simulink model "WindPrototipeN"  (R2019b)
settings: Solver=ode23s  StartTime=0.0  StopTime=Ts  FixedStep=2  RelTol=5
values from neighbouring files (symbols this model uses):
  c1 = 0.51763    [matlab.mat]
  c2 = 116    [matlab.mat]
  c3 = 0.4    [matlab.mat]
  c4 = 5    [matlab.mat]
  c5 = 21    [matlab.mat]
  c6 = 0.006795    [matlab.mat]
  Tp = 2e-05    [matlab.mat]
undefined symbols (not defined in the file or in its folder): Cogent, DiscIntNeverNeededParam, Ion, Kepware, Lithium, localhost, sigbuilder_block
libraries: powerlib x266, powerlib_extras x83, simulink x30, powerlib_meascontrol x13, opclib x11, sldrtlib x8, electricdrivelib x3
(part 7 of 9)

== system WindPrototipeN/Дом 2/ВЕТРОТУРБИНА И ГЕНЕРАТОР1/Модель турбины ==
  Generator speed (pu) : Inport
  Pitch angle (deg) : Inport  Port=2
  Wind speed (m/s) : Inport  Port=3
  Air density : Inport  Port=4
  1/cp_nom : Gain  Gain=1/cp_nom  SaturateOnIntegerOverflow=on  OutDataTypeStr=Inherit: Same as input  ParamDataTypeStr=Inherit: Same as input
  1/wind_base : Gain  Gain=1/wind_base  SaturateOnIntegerOverflow=on  OutDataTypeStr=Inherit: Same as input  ParamDataTypeStr=Inherit: Same as input
  Avoid division by zero : Saturate  UpperLimit=1e6  LowerLimit=1e-6
  "Avoid division by zero " : Saturate  UpperLimit=1e6  LowerLimit=1e-6
  Gain : Gain  Gain=-1  SaturateOnIntegerOverflow=on  OutDataTypeStr=Inherit: Same as input  ParamDataTypeStr=Inherit: Same as input
  Product : Product  Inputs=/*  SaturateOnIntegerOverflow=on  OutDataTypeStr=Inherit: Same as first input
  "Product " : Product  Inputs=3  SaturateOnIntegerOverflow=on  OutDataTypeStr=Inherit: Same as first input
  Product2 : Product  Inputs=*/  SaturateOnIntegerOverflow=on  InputSameDT=on  OutDataTypeStr=Inherit: Same as first input
  Saturation1 : Saturate  UpperLimit=inf  LowerLimit=1e-6
  Scope : Scope
  cp(lambda,beta) : Subsystem
  lambda_nom : Gain  Gain=lambda_nom  SaturateOnIntegerOverflow=on  OutDataTypeStr=Inherit: Same as input  ParamDataTypeStr=Inherit: Same as input
  pu->pu : Gain  Gain=P_wind_base*Pnom/Pelec_base  SaturateOnIntegerOverflow=on  OutDataTypeStr=Inherit: Same as input  ParamDataTypeStr=Inherit: Same as input
  "pu->pu " : Gain  Gain=1/speed_nom  SaturateOnIntegerOverflow=on  OutDataTypeStr=Inherit: Same as input  ParamDataTypeStr=Inherit: Same as input
  wind_speed^3 : Fcn  Expr=u(1)^3
  Tm (pu) : Outport  VectorParamsAs1DForOutWhenUnconnected=off
  wires:
  Pitch angle (deg)/1 -> cp(lambda,beta)/2(beta)
  pu->pu/1 -> Product2/1
  cp(lambda,beta)/1(cp) -> 1/cp_nom/1
  wind_speed^3/1 -> "Product "/1  "Pwind_pu"
  Product2/1 -> Gain/1
  Avoid division by zero/1 -> Product2/2
  Wind speed (m/s)/1 -> 1/wind_base/1
  Gain/1 -> Tm (pu)/1
  Generator speed (pu)/1 -> Avoid division by zero/1, "pu->pu "/1
  "Product "/1 -> pu->pu/1  "Pm_pu"
  lambda_nom/1 -> Saturation1/1  "lambda"
  1/cp_nom/1 -> "Product "/2  "cp_pu"
  Saturation1/1 -> cp(lambda,beta)/1(lambda), Scope/1
  Product/1 -> lambda_nom/1  "lambda_pu"
  1/wind_base/1 -> wind_speed^3/1, "Avoid division by zero "/1  "wind_speed_pu"
  "Avoid division by zero "/1 -> Product/1
  "pu->pu "/1 -> Product/2
  Air density/1 -> "Product "/3

== system WindPrototipeN/Дом 2/ВЕТРОТУРБИНА И ГЕНЕРАТОР1/Расчет номинального момента ==
  ПВ : Inport
  ОП : Inport  Port=2
  Base Torque : Product  Inputs=*/  RndMeth=Zero
  Base_torque_ : Display
  Constant1 : Constant  Value=8500
  Constant2 : Constant  Value=152.89
  Manual Switch1 : ManualSwitch  CurrentSetting=0
  Mux : Mux  Inputs=6
  Корректирующий коэффициент1 : Constant  Value=.0000133
  Коэффициент эффективности : Constant  Value=.43
  Номинальная мощность Вт : Constant  Value=2200
  Номинальная скорость ветра : Constant  Value=10
  Расчет номинального момента : Fcn  Expr=1/2*u(1)*u(2)*u(3)*u(4)^3*u(5)*u(6)
  Номинальный момент : Outport  VectorParamsAs1DForOutWhenUnconnected=off
  r : Outport  Port=2  VectorParamsAs1DForOutWhenUnconnected=off
  wires:
  Constant1/1 -> Base Torque/1
  ОП/1 -> Mux/2
  Расчет номинального момента/1 -> Manual Switch1/2, Base_torque_/1
  Коэффициент эффективности/1 -> Mux/3
  Номинальная скорость ветра/1 -> Mux/4
  Корректирующий коэффициент1/1 -> Mux/5
  Mux/1 -> Расчет номинального момента/1
  Номинальная мощность Вт/1 -> Mux/6
  Constant2/1 -> Manual Switch1/1
  Manual Switch1/1 -> r/1, Base Torque/2
  ПВ/1 -> Mux/1
  Base Torque/1 -> Номинальный момент/1

== system WindPrototipeN/Дом 2/ВХОДНЫЕ ЗНАЧЕНИЯ ДЛЯ ВЭУ1/Задание кривой скорости ==
  Demux : Demux  Tag=STV Demux  Outputs=1
  FromWs : FromWorkspace  Tag=STV FromWs  VariableName=tuvar  SampleTime=0
      SigBuilderData=|
      | common.afterFinalStr = 'Extrapolate'
      | common.sampleTime = 0
      | dataSet.timeRange = [0 15]
      | dataSet.name = 'Group 1'
      | sbobj.Groups.Name = 'Group 1'
      | sbobj.Groups.Signals.Name = 'Signal 1'
      | sbobj.Groups.Signals.XData = [0 1.5 2 2.5 3 4 4 5 5 7 8 9 11 15]
      | sbobj.Groups.Signals.YData = [8.31 8.86 8.78 8.7 7.74 8.06 8.12 7.62 7.9 7.5 7.18 7.84 7.32 6.54]
      | sbobj.Groups.TimeRange = [0 15]
  Signal 1 : Outport  Tag=STV Outport  VectorParamsAs1DForOutWhenUnconnected=off
  wires:
  Demux/1 -> Signal 1/1
  FromWs/1 -> Demux/1

== system WindPrototipeN/Дом 2/ВХОДНЫЕ ЗНАЧЕНИЯ ДЛЯ ВЭУ1/Задание кривой скорости1 ==
  Demux : Demux  Tag=STV Demux  Outputs=1
  FromWs : FromWorkspace  Tag=STV FromWs  VariableName=tuvar  SampleTime=0
      SigBuilderData=|
      | common.afterFinalStr = 'Extrapolate'
      | common.sampleTime = 0
      | dataSet.timeRange = [0 15]
      | dataSet.name = 'Group 1'
      | sbobj.Groups.Name = 'Group 1'
      | sbobj.Groups.Signals.Name = 'Signal 1'
      | sbobj.Groups.Signals.XData = [0 1.5 2 2.5 3 4 5 7 8 9 11 15]
      | sbobj.Groups.Signals.YData = [11.1 11.6 11.9 12.12 11.88 11.32 11.98 11.6 12 11.56 11.26 12]
      | sbobj.Groups.TimeRange = [0 15]
  Signal 1 : Outport  Tag=STV Outport  VectorParamsAs1DForOutWhenUnconnected=off
  wires:
  Demux/1 -> Signal 1/1
  FromWs/1 -> Demux/1

== system WindPrototipeN/Дом 2/ВХОДНЫЕ ЗНАЧЕНИЯ ДЛЯ СЭС1/Задание кривой солнечной радиации ==
  Demux : Demux  Tag=STV Demux
  FromWs : FromWorkspace  Tag=STV FromWs  VariableName=tuvar  SampleTime=0
      SigBuilderData=|
      | common.afterFinalStr = 'Extrapolate'
      | common.sampleTime = 0
      | dataSet.timeRange = [0 15]
      | dataSet.name = 'Group 1'
      | sbobj.Groups.Name = 'Group 1'
      | sbobj.Groups.Signals(1).Name = 'Signal 1'
      | sbobj.Groups.Signals(1).XData = [0 1 5 8 9 15]
      | sbobj.Groups.Signals(1).YData = [0 115 210 528 230 0]
      | sbobj.Groups.Signals(2).Name = 'Signal 2'
      | sbobj.Groups.Signals(2).XData = [0 2 2 3 3 15]
      | sbobj.Groups.Signals(2).YData = [0 0 1 1 0 0]
      | sbobj.Groups.Signals(3).Name = 'Signal 3'
      | sbobj.Groups.Signals(3).XData = [0 2.5 2.5 15]
      | sbobj.Groups.Signals(3).YData = [0 0 1 1]
      | sbobj.Groups.Signals(4).Name = 'Signal 4'
      | sbobj.Groups.Signals(4).XData = [0 2.5 2.5 15]
      | sbobj.Groups.Signals(4).YData = [0 0 1 1]
      | sbobj.Groups.TimeRange = [0 15]
  Signal 1 : Outport  Tag=STV Outport  VectorParamsAs1DForOutWhenUnconnected=off
  Signal 2 : Outport  Tag=STV Outport  Port=2
  Signal 3 : Outport  Tag=STV Outport  Port=3
  Signal 4 : Outport  Tag=STV Outport  Port=4
  wires:
  Demux/1 -> Signal 1/1
  FromWs/1 -> Demux/1
  Demux/2 -> Signal 2/1
  Demux/3 -> Signal 3/1
  Demux/4 -> Signal 4/1

== system WindPrototipeN/Дом 2/КОНТРОЛЛЕР БАТАРЕИ/Discrete PI Controller ==
  Error : Inport
  Discrete-Time Integrator : DiscreteIntegrator  InitialCondition=Init  SampleTime=Ts  LimitOutput=on  UpperSaturationLimit=UpperLimit  LowerSaturationLimit=LowerLimit  ICPrevOutput=DiscIntNeverNeededParam  ICPrevScaledInput=DiscIntNeverNeededParam
  Kp4 : Gain  Gain=Kp  SaturateOnIntegerOverflow=on  OutDataTypeStr=Inherit: Same as input  ParamDataTypeStr=Inherit: Same as input
  Kp5 : Gain  Gain=Ki  SaturateOnIntegerOverflow=on  OutDataTypeStr=Inherit: Same as input  ParamDataTypeStr=Inherit: Same as input
  Saturation2 : Saturate  UpperLimit=UpperLimit  LowerLimit=LowerLimit
  Sum6 : Sum  SaturateOnIntegerOverflow=on  InputSameDT=on  OutDataTypeStr=Inherit: Same as first input
  Out : Outport  InitialOutput=0  VectorParamsAs1DForOutWhenUnconnected=off
  wires:
  Saturation2/1 -> Out/1
  Discrete-Time Integrator/1 -> Sum6/2
  Kp4/1 -> Sum6/1
  Kp5/1 -> Discrete-Time Integrator/1
  Sum6/1 -> Saturation2/1
  Error/1 -> Kp5/1, Kp4/1

== system WindPrototipeN/Дом 2/КОНТРОЛЛЕР БАТАРЕИ/Discrete PI Controller1 ==
  Error : Inport
  Discrete-Time Integrator : DiscreteIntegrator  InitialCondition=Init  SampleTime=Ts  LimitOutput=on  UpperSaturationLimit=UpperLimit  LowerSaturationLimit=LowerLimit  ICPrevOutput=DiscIntNeverNeededParam  ICPrevScaledInput=DiscIntNeverNeededParam
  Kp4 : Gain  Gain=Kp  SaturateOnIntegerOverflow=on  OutDataTypeStr=Inherit: Same as input  ParamDataTypeStr=Inherit: Same as input
  Kp5 : Gain  Gain=Ki  SaturateOnIntegerOverflow=on  OutDataTypeStr=Inherit: Same as input  ParamDataTypeStr=Inherit: Same as input
  Saturation2 : Saturate  UpperLimit=UpperLimit  LowerLimit=LowerLimit
  Sum6 : Sum  SaturateOnIntegerOverflow=on  InputSameDT=on  OutDataTypeStr=Inherit: Same as first input
  Out : Outport  InitialOutput=0  VectorParamsAs1DForOutWhenUnconnected=off
  wires:
  Saturation2/1 -> Out/1
  Discrete-Time Integrator/1 -> Sum6/2
  Kp4/1 -> Sum6/1
  Kp5/1 -> Discrete-Time Integrator/1
  Sum6/1 -> Saturation2/1
  Error/1 -> Kp5/1, Kp4/1

== system WindPrototipeN/Дом 2/КОНТРОЛЛЕР БАТАРЕИ/Ramp_generator ==
  note: Carrier Freq
  Constant3 : Constant
  Discrete-Time Integrator1 : DiscreteIntegrator  ExternalReset=rising  SampleTime=20e-6  ICPrevOutput=DiscIntNeverNeededParam  ICPrevScaledInput=DiscIntNeverNeededParam
  Relational Operator1 : RelationalOperator  RndMeth=Nearest  InputSameDT=on
  Unit Delay1 : UnitDelay  SampleTime=20e-6  HasFrameUpgradeWarning=on
  fc : Constant  Value=10000
  ramp_out : Outport  VectorParamsAs1DForOutWhenUnconnected=off
  wires:
  Unit Delay1/1 -> Discrete-Time Integrator1/2
  Relational Operator1/1 -> Unit Delay1/1
  Constant3/1 -> Relational Operator1/2
  Discrete-Time Integrator1/1 -> ramp_out/1, Relational Operator1/1
  fc/1 -> Discrete-Time Integrator1/1

== system WindPrototipeN/Дом 2/ПОТРЕБИТЕЛЬ1/Subsystem1 ==
  Logical Operator{,1..3} (4 alike) : Logic  AllPortsSameDT=off  OutDataTypeStr=boolean
  Subsystem : Subsystem
  Кривая потребления : Subsystem  Tag=STV Subsys  LoadFcn=sigbuilder_block('load');  StartFcn=sigbuilder_block('start');  StopFcn=sigbuilder_block('stop');  ClipboardFcn=sigbuilder_block('clipboard');  mask(Sigbuilder block){tuvar=[0:10]}
      mask help: Simulink:masks:SigbuilderBlock_MD
      mask init:
      | if ~strcmp(get_param(bdroot(gcbh),'SimulationStatus'),'stopped') tuvar = sigbuilder_block('maskInit'); end
      settings: CopyFcn=sigbuilder_block('copy');  DeleteFcn=sigbuilder_block('delete');  ModelCloseFcn=sigbuilder_block('modelClose');  PreSaveFcn=sigbuilder_block('preSave');  PauseFcn=sigbuilder_block('pause');  ContinueFcn=sigbuilder_block('continue');  NameChangeFcn=sigbuilder_block('namechange');  OpenFcn=sigbuilder_block('open',[142.5 191.25 550.5 399.75 ]);  CloseFcn=sigbuilder_block('close');
      mask Display: plot(0, 0, 100, 100,[2, 2, 32, 32, 2], [68, 8, 8, 68, 68],[32, 2], [38, 38], [32, 19, 2],[53, 60, 44], [32, 17, 17, 2],[16, 16, 31, 31]);txt = getActiveGroup(gcbh);text(2, 100, txt,'verticalAlignment', 'top');
  Out1 : Outport
  Out2 : Outport  Port=2
  Out3 : Outport  Port=3
  Out4 : Outport  Port=4
  wires:
  Кривая потребления/4(Signal 4) -> Logical Operator3/2
  Subsystem/2(Out2) -> Logical Operator1/1
  Logical Operator/1 -> Out1/1
  Subsystem/4(Out4) -> Logical Operator3/1
  Subsystem/1(Out1) -> Logical Operator/1
  Кривая потребления/1(Signal 2) -> Logical Operator/2
  Кривая потребления/2(Signal 1) -> Logical Operator1/2
  Logical Operator2/1 -> Out3/1
  Кривая потребления/3(Signal 3) -> Logical Operator2/2
  Subsystem/3(Out3) -> Logical Operator2/1
  Logical Operator1/1 -> Out2/1
  Logical Operator3/1 -> Out4/1

== system WindPrototipeN/Дом 2/СОЛНЕЧНЫЕ ПАНЕЛИ1/11*2=666 V ==
  In1 : Inport
  Solar : Subsystem
  Conn1 : PMIOPort  Side=Right
  Conn2 : PMIOPort  Port=2  Side=Right
  wires:
  In1/1 -> Solar/1(In1)
  connections:
  Solar/RConn1 -- Conn1/RConn1
  Solar/RConn3 -- Solar/RConn2
  Conn2/RConn1 -- Solar/RConn4

== system WindPrototipeN/Дом 3/DC//AC 220В1/LC Фильтр ==
  "2 mH " : powerlib/Elements/Three-Phase Series RLC Branch  LConnTagsString=A|B|C  RConnTagsString=A|B|C  BranchType=L  Resistance=1.0  Inductance=36e-4  Capacitance=1.0  Measurements=None
      settings: SourceProductName=Simscape Electrical
  Ground : powerlib/Elements/Ground  LConnTagsString=a
      settings: SourceProductName=Simscape Electrical
  Ground1 : powerlib/Elements/Ground  LConnTagsString=a
      settings: SourceProductName=Simscape Electrical
  Ground2 : powerlib/Elements/Ground  LConnTagsString=a
      settings: SourceProductName=Simscape Electrical
  Three-Phase Series RLC Branch : powerlib/Elements/Three-Phase Series RLC Branch  LConnTagsString=A|B|C  RConnTagsString=A|B|C  BranchType=C  Resistance=.1  Inductance=1e-3  Capacitance=6.85e-6  Measurements=None
      settings: SourceProductName=Simscape Electrical
  A : PMIOPort  Side=Left
  B : PMIOPort  Port=2  Side=Left
  C : PMIOPort  Port=3  Side=Left
  "A " : PMIOPort  Port=4  Side=Right
  "B " : PMIOPort  Port=5  Side=Right
  "C " : PMIOPort  Port=6  Side=Right
  connections:
  B/RConn1 -- "2 mH "/LConn2
  A/RConn1 -- "2 mH "/LConn1
  C/RConn1 -- "2 mH "/LConn3
  "2 mH "/RConn1 -- "A "/RConn1 -- Three-Phase Series RLC Branch/LConn1
  "2 mH "/RConn2 -- "B "/RConn1 -- Three-Phase Series RLC Branch/LConn2
  "2 mH "/RConn3 -- "C "/RConn1 -- Three-Phase Series RLC Branch/LConn3
  Ground/LConn1 -- Three-Phase Series RLC Branch/RConn1
  Ground1/LConn1 -- Three-Phase Series RLC Branch/RConn2
  Ground2/LConn1 -- Three-Phase Series RLC Branch/RConn3

== system WindPrototipeN/Дом 3/DC//AC 220В1/Инвертор DC//AC ==
  Discrete PWM Generator1 : Subsystem  AncestorBlock=|  DialogController=POWERSYS.PowerSysDialog  mask(Discrete PWM Generator){GeneratorMode=3-arm  bridge (6 pulses), Fc=4000, Ts=20e-6, Internal=off, mIndex=0.4, Freq=60, Phase=0}
      | powerlib_extras/Discrete 
      | Control Blocks/Discrete
      | PWM Generator
      mask prompts: GeneratorMode "Generator Mode"; Fc "Carrier frequency (Hz):"; Ts "Sample time:"; Internal "Internal generation of modulating signal(s)"; mIndex "Modulation index  (0<m<1) :"; Freq "Frequency of output voltage (Hz)"; Phase "Phase of output voltage (degrees)"
      mask help:
      | This discrete block generates pulses for carrier-based PWM (Pulse Width Modulation), self-commutated IGBTs,GTOs or FETs bridges.
      |
      | Depending on the number of bridge arms selected in the "Generator Mode" parameter, the block can be used either for single-phase or three-phase PWM control.
      mask init: same as WindPrototipeN/Дом 1/DC//AC 220В/Инвертор DC//AC/Discrete PWM Generator1
      mask Help:
      | The output pulses are a vector (with values=0 or 1). Depending on the selected "Generator Mode", the output vector contains:
      | For a 1-arm  bridge: Two pulses. Pulse 1 is for the upper switch and pulse 2 is for the lower switch.
      | For a 2-arm  bridge: Four pulses. Pulses 1 and 3 are respectively for the upper switches of the first and second arm. Pulses 2 and 4 are for the lower switches.
      | For a 3-arm  bridge: Six pulses. Pulses 1,3 and 5 are respectively for the upper switches of the first,second and third arm. Pulses 2,4 and 6 are for the lower switches.
      | For double 3-arm bridges: Twelve pulses.The first six pulses (pulses 1 to 6) must be sent to the first 3-arm bridge and the last six (pulses 7 to 12) to the second 3-arm bridge.
      | 
      | By selecting "Internal generation" you can can control the modulation index m, frequency and phase of the output voltage  from the internal parameters (m, Freq and Phase). Otherwise, external signals are used for pulse generation. The width of the input vector must be 1 for single phase bridges ( 1-arm or 2-arm)  and 3 for 3-phase bridges  (single or double bridge).
      mask TypeOptions GeneratorMode: 1-arm  bridge (2 pulses) | 2-arm  bridge (4 pulses) | 3-arm  bridge (6 pulses) | Double 3-arm  bridges (12 pulses)
      mask Callback Internal: powericon('psbcallbacks',gcb,'Discrete PWM Generator',[]);
  MI Controller : Subsystem
  Subsystem1 : Subsystem
  Unit Delay4 : UnitDelay  SampleTime=20e-6  HasFrameUpgradeWarning=on
  C : PMIOPort  Side=Left
  B : PMIOPort  Port=2  Side=Left
  A : PMIOPort  Port=3  Side=Left
  VL : Outport  VectorParamsAs1DForOutWhenUnconnected=off
  Vp : Outport  Port=2  VectorParamsAs1DForOutWhenUnconnected=off
  Pulses : Outport  Port=3  VectorParamsAs1DForOutWhenUnconnected=off
  wires:
  Unit Delay4/1 -> Pulses/1
  Discrete PWM Generator1/1(Pulses) -> Unit Delay4/1
  MI Controller/1(Vabc_inv) -> Discrete PWM Generator1/1(Uref)
  Subsystem1/1(Vph) -> MI Controller/1(Vabc)
  Subsystem1/2(VL-L) -> VL/1
  Subsystem1/3(Vph_rms) -> Vp/1
  connections:
  A/RConn1 -- Subsystem1/LConn1
  B/RConn1 -- Subsystem1/LConn2
  C/RConn1 -- Subsystem1/LConn3

== system WindPrototipeN/Дом 3/DC//DC ПРЕОБРАЗОВАТЕЛЬ ВЭУ1/Chopper ==
  Duty Cycle : Inport
  Average-value armature voltage : Fcn  Expr=u(1)*u(2)
  Average-value source current : Fcn  Expr=u(1)*u(2)
  Controlled Current Source : powerlib/Electrical Sources/Controlled Current Source  Initialize=on  Source_Type=AC  Amplitude=0  Phase=0  Frequency=0  Measurements=None
      settings: SourceProductName=Simscape Electrical
  Controlled Voltage Source : powerlib/Electrical Sources/Controlled Voltage Source  Initialize=on  Source_Type=AC  Amplitude=0  Phase=0  Frequency=0  Measurements=None
      settings: SourceProductName=Simscape Electrical
  Current Measurement : powerlib/Measurements/Current Measurement  Tag=PoWeRsYsTeMmEaSuReMeNt  PhasorSimulation=off  OutputType=Magnitude  PSBequivalent=0
      settings: SourceProductName=Simscape Electrical
  Memory : Memory
  Memory1 : Memory
  Mux : Mux  Inputs=2
  Mux1 : Mux  Inputs=2
  Selector : Selector  InputPortWidth=2  IndexOptions=Index vector (dialog)  Indices=[1]  OutputSizes=1
  Voltage Measurement1 : powerlib/Measurements/Voltage Measurement  Tag=PoWeRsYsTeMmEaSuReMeNt  PhasorSimulation=off  OutputType=Magnitude  PSBequivalent=0
      settings: SourceProductName=Simscape Electrical
  A : PMIOPort  Side=Right
  + : PMIOPort  Port=2  Side=Left
  - : PMIOPort  Port=3  Side=Left
  wires:
  Memory/1 -> Controlled Voltage Source/1
  Average-value armature voltage/1 -> Memory/1
  Mux/1 -> Average-value armature voltage/1
  Voltage Measurement1/1 -> Mux/2
  Duty Cycle/1 -> Selector/1
  Mux1/1 -> Average-value source current/1
  Current Measurement/1 -> Mux1/2
  Average-value source current/1 -> Memory1/1
  Memory1/1 -> Controlled Current Source/1
  Selector/1 -> Mux/1, Mux1/1
  connections:
  Voltage Measurement1/LConn2 -- Controlled Current Source/RConn1 -- -/RConn1 -- Controlled Voltage Source/LConn1
  Controlled Current Source/LConn1 -- Voltage Measurement1/LConn1 -- +/RConn1
  Controlled Voltage Source/RConn1 -- Current Measurement/LConn1
  A/RConn1 -- Current Measurement/RConn1

== system WindPrototipeN/Дом 3/DC//DC ПРЕОБРАЗОВАТЕЛЬ ВЭУ1/Current controller DISCRETE1 ==
  UBus : Inport
  Uref : Inport  Port=2
  Ctrl sat. : Saturate  UpperLimit=0.95  LowerLimit=-0.95
  Discrete-Time Integrator : DiscreteIntegrator  IntegratorMethod=Integration: Trapezoidal  SampleTime=Ts  LimitOutput=on  UpperSaturationLimit=0.95  LowerSaturationLimit=-0.95  ICPrevOutput=DiscIntNeverNeededParam  ICPrevScaledInput=DiscIntNeverNeededParam
  Integral gain : Gain  Gain=Ki  SaturateOnIntegerOverflow=on  OutDataTypeStr=Inherit: Same as input  ParamDataTypeStr=Inherit: Same as input
  Proportional gain : Gain  Gain=Kp  SaturateOnIntegerOverflow=on  OutDataTypeStr=Inherit: Same as input  ParamDataTypeStr=Inherit: Same as input
  Sum1 : Sum  Inputs=+-  SaturateOnIntegerOverflow=on  InputSameDT=on  OutDataTypeStr=Inherit: Same as first input
  Sum2 : Sum  SaturateOnIntegerOverflow=on  InputSameDT=on  OutDataTypeStr=Inherit: Same as first input
  Ec : Outport  InitialOutput=0  VectorParamsAs1DForOutWhenUnconnected=off
  wires:
  Proportional gain/1 -> Sum2/1
  Integral gain/1 -> Discrete-Time Integrator/1
  Sum1/1 -> Integral gain/1, Proportional gain/1
  UBus/1 -> Sum1/1
  Uref/1 -> Sum1/2
  Discrete-Time Integrator/1 -> Sum2/2
  Sum2/1 -> Ctrl sat./1
  Ctrl sat./1 -> Ec/1

== system WindPrototipeN/Дом 3/DC//DC ПРЕОБРАЗОВАТЕЛЬ ВЭУ1/Current controller DISCRETE2 ==
  Pref : Inport
  Ppv : Inport  Port=2
  Ctrl sat. : Saturate  UpperLimit=0.95  LowerLimit=-0.95
  Discrete-Time Integrator : DiscreteIntegrator  IntegratorMethod=Integration: Trapezoidal  SampleTime=Ts  LimitOutput=on  UpperSaturationLimit=0.95  LowerSaturationLimit=-0.95  ICPrevOutput=DiscIntNeverNeededParam  ICPrevScaledInput=DiscIntNeverNeededParam
  Integral gain : Gain  Gain=Ki  SaturateOnIntegerOverflow=on  OutDataTypeStr=Inherit: Same as input  ParamDataTypeStr=Inherit: Same as input
  Proportional gain : Gain  Gain=Kp  SaturateOnIntegerOverflow=on  OutDataTypeStr=Inherit: Same as input  ParamDataTypeStr=Inherit: Same as input
  Sum1 : Sum  Inputs=+-  SaturateOnIntegerOverflow=on  InputSameDT=on  OutDataTypeStr=Inherit: Same as first input
  Sum2 : Sum  SaturateOnIntegerOverflow=on  InputSameDT=on  OutDataTypeStr=Inherit: Same as first input
  Delta Ec : Outport  InitialOutput=0  VectorParamsAs1DForOutWhenUnconnected=off
  wires:
  Ctrl sat./1 -> Delta Ec/1
  Sum2/1 -> Ctrl sat./1
  Discrete-Time Integrator/1 -> Sum2/2
  Ppv/1 -> Sum1/2
  Pref/1 -> Sum1/1
  Sum1/1 -> Proportional gain/1, Integral gain/1
  Integral gain/1 -> Discrete-Time Integrator/1
  Proportional gain/1 -> Sum2/1

== system WindPrototipeN/Дом 3/DC//DC ПРЕОБРАЗОВАТЕЛЬ ВЭУ1/Duty Cycles ==
  Ec : Inport
  Add : Sum  Inputs=+-
  Bus Creator2 : BusCreator  Inputs=2
  Constant : Constant
  Duty Cycle : Fcn  Expr=0.5*(u[1]+1)
  dc : Outport  VectorParamsAs1DForOutWhenUnconnected=off
  wires:
  Duty Cycle/1 -> Add/2, Bus Creator2/1  "IGBT I"
  Add/1 -> Bus Creator2/2  "IGBT 2"
  Constant/1 -> Add/1
  Ec/1 -> Duty Cycle/1
  Bus Creator2/1 -> dc/1

== system WindPrototipeN/Дом 3/DC//DC ПРЕОБРАЗОВАТЕЛЬ ВЭУ1/Timer ==
  Clock : Clock
  Derivative : Derivative
  Hit Crossing : HitCross  ShowOutputPort=off
  Look-Up Table : Lookup  InputValues=tv  Table=opv  SaturateOnIntegerOverflow=on
  Out : Outport  VectorParamsAs1DForOutWhenUnconnected=off
  wires:
  Clock/1 -> Look-Up Table/1
  Look-Up Table/1 -> Out/1, Derivative/1
  Derivative/1 -> Hit Crossing/1

== system WindPrototipeN/Дом 3/DC//DC ПРЕОБРАЗОВАТЕЛЬ СП1/Chopper ==
  Duty Cycle : Inport
  Average-value armature voltage : Fcn  Expr=u(1)*u(2)
  Average-value source current : Fcn  Expr=u(1)*u(2)
  Controlled Current Source : powerlib/Electrical Sources/Controlled Current Source  Initialize=on  Source_Type=AC  Amplitude=0  Phase=0  Frequency=0  Measurements=None
      settings: SourceProductName=Simscape Electrical
  Controlled Voltage Source : powerlib/Electrical Sources/Controlled Voltage Source  Initialize=on  Source_Type=AC  Amplitude=0  Phase=0  Frequency=0  Measurements=None
      settings: SourceProductName=Simscape Electrical
  Current Measurement : powerlib/Measurements/Current Measurement  Tag=PoWeRsYsTeMmEaSuReMeNt  PhasorSimulation=off  OutputType=Magnitude  PSBequivalent=0
      settings: SourceProductName=Simscape Electrical
  Memory : Memory
  Memory1 : Memory
  Mux : Mux  Inputs=2
  Mux1 : Mux  Inputs=2
  Selector : Selector  InputPortWidth=2  IndexOptions=Index vector (dialog)  Indices=[1]  OutputSizes=1
  Voltage Measurement1 : powerlib/Measurements/Voltage Measurement  Tag=PoWeRsYsTeMmEaSuReMeNt  PhasorSimulation=off  OutputType=Magnitude  PSBequivalent=0
      settings: SourceProductName=Simscape Electrical
  A : PMIOPort  Side=Right
  + : PMIOPort  Port=2  Side=Left
  - : PMIOPort  Port=3  Side=Left
  wires:
  Memory/1 -> Controlled Voltage Source/1
  Average-value armature voltage/1 -> Memory/1
  Mux/1 -> Average-value armature voltage/1
  Voltage Measurement1/1 -> Mux/2
  Duty Cycle/1 -> Selector/1
  Mux1/1 -> Average-value source current/1
  Current Measurement/1 -> Mux1/2
  Average-value source current/1 -> Memory1/1
  Memory1/1 -> Controlled Current Source/1
  Selector/1 -> Mux/1, Mux1/1
  connections:
  Voltage Measurement1/LConn2 -- Controlled Current Source/RConn1 -- -/RConn1 -- Controlled Voltage Source/LConn1
  Controlled Current Source/LConn1 -- Voltage Measurement1/LConn1 -- +/RConn1
  Controlled Voltage Source/RConn1 -- Current Measurement/LConn1
  A/RConn1 -- Current Measurement/RConn1

== system WindPrototipeN/Дом 3/DC//DC ПРЕОБРАЗОВАТЕЛЬ СП1/Current controller DISCRETE1 ==
  UBus : Inport
  Uref : Inport  Port=2
  Ctrl sat. : Saturate  UpperLimit=0.95  LowerLimit=-0.95
  Discrete-Time Integrator : DiscreteIntegrator  IntegratorMethod=Integration: Trapezoidal  SampleTime=Ts  LimitOutput=on  UpperSaturationLimit=0.95  LowerSaturationLimit=-0.95  ICPrevOutput=DiscIntNeverNeededParam  ICPrevScaledInput=DiscIntNeverNeededParam
  Integral gain : Gain  Gain=Ki  SaturateOnIntegerOverflow=on  OutDataTypeStr=Inherit: Same as input  ParamDataTypeStr=Inherit: Same as input
  Proportional gain : Gain  Gain=Kp  SaturateOnIntegerOverflow=on  OutDataTypeStr=Inherit: Same as input  ParamDataTypeStr=Inherit: Same as input
  Sum1 : Sum  Inputs=+-  SaturateOnIntegerOverflow=on  InputSameDT=on  OutDataTypeStr=Inherit: Same as first input
  Sum2 : Sum  SaturateOnIntegerOverflow=on  InputSameDT=on  OutDataTypeStr=Inherit: Same as first input
  Ec : Outport  InitialOutput=0  VectorParamsAs1DForOutWhenUnconnected=off
  wires:
  Proportional gain/1 -> Sum2/1
  Integral gain/1 -> Discrete-Time Integrator/1
  Sum1/1 -> Integral gain/1, Proportional gain/1
  UBus/1 -> Sum1/1
  Uref/1 -> Sum1/2
  Discrete-Time Integrator/1 -> Sum2/2
  Sum2/1 -> Ctrl sat./1
  Ctrl sat./1 -> Ec/1

== system WindPrototipeN/Дом 3/DC//DC ПРЕОБРАЗОВАТЕЛЬ СП1/Current controller DISCRETE2 ==
  Pref : Inport
  Ppv : Inport  Port=2
  Ctrl sat. : Saturate  UpperLimit=0.95  LowerLimit=-0.95
  Discrete-Time Integrator : DiscreteIntegrator  IntegratorMethod=Integration: Trapezoidal  SampleTime=Ts  LimitOutput=on  UpperSaturationLimit=0.95  LowerSaturationLimit=-0.95  ICPrevOutput=DiscIntNeverNeededParam  ICPrevScaledInput=DiscIntNeverNeededParam
  Integral gain : Gain  Gain=Ki  SaturateOnIntegerOverflow=on  OutDataTypeStr=Inherit: Same as input  ParamDataTypeStr=Inherit: Same as input
  Proportional gain : Gain  Gain=Kp  SaturateOnIntegerOverflow=on  OutDataTypeStr=Inherit: Same as input  ParamDataTypeStr=Inherit: Same as input
  Sum1 : Sum  Inputs=+-  SaturateOnIntegerOverflow=on  InputSameDT=on  OutDataTypeStr=Inherit: Same as first input
  Sum2 : Sum  SaturateOnIntegerOverflow=on  InputSameDT=on  OutDataTypeStr=Inherit: Same as first input
  Delta Ec : Outport  InitialOutput=0  VectorParamsAs1DForOutWhenUnconnected=off
  wires:
  Ctrl sat./1 -> Delta Ec/1
  Sum2/1 -> Ctrl sat./1
  Discrete-Time Integrator/1 -> Sum2/2
  Ppv/1 -> Sum1/2
  Pref/1 -> Sum1/1
  Sum1/1 -> Proportional gain/1, Integral gain/1
  Integral gain/1 -> Discrete-Time Integrator/1
  Proportional gain/1 -> Sum2/1

== system WindPrototipeN/Дом 3/DC//DC ПРЕОБРАЗОВАТЕЛЬ СП1/Duty Cycles ==
  Ec : Inport
  Add : Sum  Inputs=+-
  Bus Creator2 : BusCreator  Inputs=2
  Constant : Constant
  Duty Cycle : Fcn  Expr=0.5*(u[1]+1)
  dc : Outport  VectorParamsAs1DForOutWhenUnconnected=off
  wires:
  Duty Cycle/1 -> Add/2, Bus Creator2/1  "IGBT I"
  Add/1 -> Bus Creator2/2  "IGBT 2"
  Constant/1 -> Add/1
  Ec/1 -> Duty Cycle/1
  Bus Creator2/1 -> dc/1

== system WindPrototipeN/Дом 3/DC//DC ПРЕОБРАЗОВАТЕЛЬ СП1/Timer ==
  Clock : Clock
  Derivative : Derivative
  Hit Crossing : HitCross  ShowOutputPort=off
  Look-Up Table : Lookup  InputValues=tv  Table=opv  SaturateOnIntegerOverflow=on
  Out : Outport  VectorParamsAs1DForOutWhenUnconnected=off
  wires:
  Clock/1 -> Look-Up Table/1
  Look-Up Table/1 -> Out/1, Derivative/1
  Derivative/1 -> Hit Crossing/1

== system WindPrototipeN/Дом 3/MPPT КОНТРОЛЛЕР МОЩНОСТИ ВЭУ1/Контроллер силы тока ==
  Iref : Inport
  Ia : Inport  Port=2
  Relay : Relay  OnSwitchValue=h/2  OffSwitchValue=-h/2
  Sum1 : Sum  Inputs=-+  SaturateOnIntegerOverflow=on  InputSameDT=on  OutDataTypeStr=Inherit: Same as first input
  g : Outport  InitialOutput=0  VectorParamsAs1DForOutWhenUnconnected=off
  error1 : Outport  Port=2  InitialOutput=0  VectorParamsAs1DForOutWhenUnconnected=off
  wires:
  Relay/1 -> g/1
  Ia/1 -> Sum1/1
  Iref/1 -> Sum1/2
  Sum1/1 -> Relay/1, error1/1

== system WindPrototipeN/Дом 3/MPPT КОНТРОЛЛЕР МОЩНОСТИ ВЭУ1/Расчет опорного момента ==
  wm : Inport
  Constant2 : Constant  Value=1.791e-3
  Math Function : Math  Operator=square  SaturateOnIntegerOverflow=on
  Product1 : Product  RndMeth=Zero
  Ref. sat.1 : Saturate  UpperLimit=inf  LowerLimit=0
  Tref : Outport  VectorParamsAs1DForOutWhenUnconnected=off
  wires:
  Math Function/1 -> Product1/1
  Constant2/1 -> Product1/2
  wm/1 -> Math Function/1
  Ref. sat.1/1 -> Tref/1
  Product1/1 -> Ref. sat.1/1

== system WindPrototipeN/Дом 3/MPPT КОНТРОЛЛЕР МОЩНОСТИ ВЭУ1/Расчет опорной силы тока ==
  Tref : Inport
  wm : Inport  Port=2
  Vd : Inport  Port=3
  Avoid division by zero : Saturate  UpperLimit=1e6  LowerLimit=1e-6
  Base Torque1 : Product  Inputs=*/  RndMeth=Zero
  Product1 : Product  RndMeth=Zero
  Scope : Scope
  Id_ref : Outport  VectorParamsAs1DForOutWhenUnconnected=off
  wires:
  Product1/1 -> Scope/1, Base Torque1/1
  Avoid division by zero/1 -> Base Torque1/2
  Tref/1 -> Product1/1
  wm/1 -> Product1/2
  Base Torque1/1 -> Id_ref/1
  Vd/1 -> Avoid division by zero/1

== system WindPrototipeN/Дом 3/ВЕТРОТУРБИНА И ГЕНЕРАТОР1/DC//DC Преобразователь (Rectifier) ==
  note: out 5
  C1 : powerlib/Elements/Parallel RLC Branch  LConnTagsString=a  RConnTagsString=__new0  BranchType=C  Resistance=1.0  Inductance=1.0  SetiL0=off  InitialCurrent=0  Capacitance=1000e-06  Setx0=off  InitialVoltage=650  Measurements=None
      settings: SourceProductName=Simscape Electrical
  C3 : powerlib/Measurements/Current Measurement  PhasorSimulation=off  OutputType=Complex  PSBequivalent=0
      settings: SourceProductName=Simscape Electrical
  Dis : powerlib_extras/Discrete  Control Blocks/Discrete 1st-Order Filter  FilterType=Lowpass  Tc=100e-3  Ts=20e-6  Initialize=off  Vac_Init=[0.8 -25 60]  Vdc_Init=-0.4  PlotResponse=off  param1=[1 500 0.1]
      settings: SourceProductName=Simscape Electrical  SourceProductBaseCode=PS
  L1 : powerlib/Elements/Series RLC Branch  LConnTagsString=__new0  RConnTagsString=__new0  BranchType=L  Resistance=1.0  Inductance=2e-3  SetiL0=off  InitialCurrent=0  Capacitance=1.0  Setx0=off  InitialVoltage=0  Measurements=None
      settings: SourceProductName=Simscape Electrical
  L2 : powerlib/Elements/Series RLC Branch  LConnTagsString=__new0  RConnTagsString=__new0  BranchType=L  Resistance=1.0  Inductance=2e-3  SetiL0=off  InitialCurrent=0  Capacitance=1.0  Setx0=off  InitialVoltage=0  Measurements=None
      settings: SourceProductName=Simscape Electrical
  Rectifier : powerlib/Power Electronics/Universal Bridge  Arms=3  SnubberResistance=100  SnubberCapacitance=0.1e-6  Device=Diodes  Ron=1e-3  Lon=0  ForwardVoltages="[  0.8  0.8  ]"  ForwardVoltage=.8  GTOparameters=[ 10e-6 , 20e-6 ]  IGBTparameters=[ 1e-6 , 2e-6 ]  Measurements=Device currents  Measurements_2=None  converterType=Rectifier
      settings: SourceProductName=Simscape Electrical
  Vdc1 : powerlib/Measurements/Voltage Measurement  Tag=PoWeRsYsTeMmEaSuReMeNt  PhasorSimulation=off  OutputType=Magnitude  PSBequivalent=0
      settings: SourceProductName=Simscape Electrical
  + : PMIOPort  Tag=PMCPort  Side=Right
  Conn2 : PMIOPort  Port=2  Side=Left
  Conn3 : PMIOPort  Port=3  Side=Left
  Conn4 : PMIOPort  Port=4  Side=Left
  - : PMIOPort  Tag=PMCPort  Port=5  Side=Right
  Id : Outport  VectorParamsAs1DForOutWhenUnconnected=off
  Vd : Outport  Port=2  VectorParamsAs1DForOutWhenUnconnected=off
  wires:
  Dis/1 -> Id/1
  Vdc1/1 -> Vd/1
  C3/1 -> Dis/1
  connections:
  C3/LConn1 -- Vdc1/LConn1 -- C1/LConn1 -- L2/RConn1
  C1/RConn1 -- -/RConn1 -- Rectifier/RConn2 -- Vdc1/LConn2
  C3/RConn1 -- L1/LConn1
  L2/LConn1 -- Rectifier/RConn1
  Conn4/RConn1 -- Rectifier/LConn3
  L1/RConn1 -- +/RConn1
  Rectifier/LConn2 -- Conn3/RConn1
  Conn2/RConn1 -- Rectifier/LConn1

== system WindPrototipeN/Дом 3/ВЕТРОТУРБИНА И ГЕНЕРАТОР1/Контроллер угла поворота ==
  wd : Inport
  P : Inport  Port=2
  0-pitch_max : Saturate  UpperLimit=54  LowerLimit=0
  Add : Sum  Inputs=|-+
  Add1 : Sum  Inputs=|+-
  Add2 : Sum  Inputs=|-+
  Constant : Constant  Value=1500
  D_power : Constant  Value=0.2
  Data Type Conversion : DataTypeConversion  OutDataTypeStr=double  RndMeth=Round
  I_gen : Constant  Value=2
  I_power : Constant  Value=10
  Mux : Mux  Inputs=2
  N_power : Constant  Value=100
  PID_power : simulink/Continuous/PID Controller  Controller=PID  Form=Parallel  TimeDomain=Discrete-time  SampleTime=20e-6  IntegratorMethod=Forward Euler  FilterMethod=Forward Euler  ControllerParametersSource=external  P=1  I=1  D=0  UseFilter=on  N=100  TunerSelectOption=Transfer Function Based (PID Tuner App)  InitialConditionSource=internal  InitialConditionForIntegrator=0  InitialConditionForFilter=0  DifferentiatorICPrevScaledInput=0  ExternalReset=none  TrackingMode=off  Kt=1  LimitOutput=on  UpperSaturationLimit=25  LowerSaturationLimit=0  LinearizeAsGain=on  AntiWindupMode=none  Kb=1  POutMin=[]  POutMax=[]  IOutMin=[]  IOutMax=[]  DOutMin=[]  DOutMax=[]  NOutMin=[]  NOutMax=[]  SumOutMin=[]  SumOutMax=[]  SaturationOutMin=[]  SaturationOutMax=[]  PParamMin=[]  PParamMax=[]  IParamMin=[]  IParamMax=[]  DParamMin=[]  DParamMax=[]  NParamMin=[]  NParamMax=[]  KbParamMin=[]  KbParamMax=[]  KtParamMin=[]  KtParamMax=[]  KbOutMin=[]  KbOutMax=[]  KtOutMin=[]  KtOutMax=[]  IntegratorOutMin=[]  IntegratorOutMax=[]  FilterOutMin=[]  FilterOutMax=[]  SumI1OutMin=[]  SumI1OutMax=[]  SumI2OutMin=[]  SumI2OutMax=[]  SumI3OutMin=[]  SumI3OutMax=[]  SumI4OutMin=[]  SumI4OutMax=[]  SumDOutMin=[]  SumDOutMax=[]  DifferentiatorOutMin=[]  DifferentiatorOutMax=[]  FilterDiffOutCoefMin=[]  FilterDiffOutCoefMax=[]  ReciprocalOutMin=[]  ReciprocalOutMax=[]  SumDenOutMin=[]  SumDenOutMax=[]  SumNumOutMin=[]  SumNumOutMax=[]  DivideOutMin=[]  DivideOutMax=[]  IntegratorContinuousStateAttributes=''  IntegratorStateMustResolveToSignalObject=off  IntegratorRTWStateStorageClass=Auto  FilterContinuousStateAttributes=''  FilterStateMustResolveToSignalObject=off  FilterRTWStateStorageClass=Auto  ParallelPVariant=ExternalParameters  IdealPVariant=Disabled  IVariant=ExternalParameters  DVariant=ExternalParameters  IntegratorVariant=Discrete  SatVariant=Enabled  AWVariant=Passthrough  PCopyVariant=Disabled  TRVariant=Disabled  FdbkBlocksVariant=Forward  IdealPFdbkVariant=Disabled  SatFdbkVariant=Disabled  DerivativeFilterVariant=ForwardEulerFilter  NVariant=ExternalParameters  NCopyVariant=Disabled  FilterICVariant=InternalICsFilter  IntegratorICVariant=InternalICs  ExternalResetVariant=Disabled  TRSumVariant=Passthrough  SumFdbkVariant=Disabled  SumVariant=Sum_PID
  PI_gen : simulink/Continuous/PID Controller  Controller=PI  Form=Parallel  TimeDomain=Discrete-time  SampleTime=20e-6  IntegratorMethod=Forward Euler  FilterMethod=Forward Euler  ControllerParametersSource=external  P=1  I=1  D=0  UseFilter=on  N=100  TunerSelectOption=Transfer Function Based (PID Tuner App)  InitialConditionSource=internal  InitialConditionForIntegrator=0  InitialConditionForFilter=0  DifferentiatorICPrevScaledInput=0  ExternalReset=none  TrackingMode=off  Kt=1  LimitOutput=on  UpperSaturationLimit=29  LowerSaturationLimit=-29  LinearizeAsGain=on  AntiWindupMode=none  Kb=1  POutMin=[]  POutMax=[]  IOutMin=[]  IOutMax=[]  DOutMin=[]  DOutMax=[]  NOutMin=[]  NOutMax=[]  SumOutMin=[]  SumOutMax=[]  SaturationOutMin=[]  SaturationOutMax=[]  PParamMin=[]  PParamMax=[]  IParamMin=[]  IParamMax=[]  DParamMin=[]  DParamMax=[]  NParamMin=[]  NParamMax=[]  KbParamMin=[]  KbParamMax=[]  KtParamMin=[]  KtParamMax=[]  KbOutMin=[]  KbOutMax=[]  KtOutMin=[]  KtOutMax=[]  IntegratorOutMin=[]  IntegratorOutMax=[]  FilterOutMin=[]  FilterOutMax=[]  SumI1OutMin=[]  SumI1OutMax=[]  SumI2OutMin=[]  SumI2OutMax=[]  SumI3OutMin=[]  SumI3OutMax=[]  SumI4OutMin=[]  SumI4OutMax=[]  SumDOutMin=[]  SumDOutMax=[]  DifferentiatorOutMin=[]  DifferentiatorOutMax=[]  FilterDiffOutCoefMin=[]  FilterDiffOutCoefMax=[]  ReciprocalOutMin=[]  ReciprocalOutMax=[]  SumDenOutMin=[]  SumDenOutMax=[]  SumNumOutMin=[]  SumNumOutMax=[]  DivideOutMin=[]  DivideOutMax=[]  IntegratorContinuousStateAttributes=''  IntegratorStateMustResolveToSignalObject=off  IntegratorRTWStateStorageClass=Auto  FilterContinuousStateAttributes=''  FilterStateMustResolveToSignalObject=off  FilterRTWStateStorageClass=Auto  ParallelPVariant=ExternalParameters  IdealPVariant=Disabled  IVariant=ExternalParameters  DVariant=Disabled  IntegratorVariant=Discrete  SatVariant=Enabled  AWVariant=Passthrough  PCopyVariant=Disabled  TRVariant=Disabled  FdbkBlocksVariant=Forward  IdealPFdbkVariant=Disabled  SatFdbkVariant=Disabled  DerivativeFilterVariant=Disabled  NVariant=Disabled  NCopyVariant=Disabled_SignalSpec  FilterICVariant=Disabled  IntegratorICVariant=InternalICs  ExternalResetVariant=Disabled  TRSumVariant=Passthrough  SumFdbkVariant=Disabled  SumVariant=Sum_PI
  P_gen : Constant  Value=70
  P_power : Constant  Value=50
  wr : Constant  Value=0.4
  График ошибки : Scope
  Ошибка ген : Display
  Ошибка мощность : Display
  Сигнал ПИ : Display
  Сигнал ПИД : Display
  Терминал ПИ : Scope  NumInputPorts=2
  Терминал ПИД : Scope  NumInputPorts=2
  Угол поворота : Display
  beta : Outport  VectorParamsAs1DForOutWhenUnconnected=off
  wires:
  wd/1 -> Add/1
  wr/1 -> Add/2
  Add/1 -> Ошибка ген/1, PI_gen/1
  P/1 -> Mux/2, Add1/1
  Constant/1 -> Mux/1, Add1/2
  Add1/1 -> Ошибка мощность/1, PID_power/1
  PI_gen/1 -> Add2/1, Сигнал ПИ/1
  PID_power/1 -> Add2/2, Сигнал ПИД/1
  [WindSpeed_ex_2] -> Терминал ПИД/2
  Mux/1 -> Терминал ПИД/1
  Data Type Conversion/1 -> beta/1, Угол поворота/1
  P_gen/1 -> PI_gen/2
  I_gen/1 -> PI_gen/3
  N_power/1 -> PID_power/5
  P_power/1 -> PID_power/2
  I_power/1 -> PID_power/3
  D_power/1 -> PID_power/4
  0-pitch_max/1 -> Терминал ПИ/1, Data Type Conversion/1, Терминал ПИ/2
  Add2/1 -> 0-pitch_max/1, График ошибки/1

== system WindPrototipeN/Дом 3/ВЕТРОТУРБИНА И ГЕНЕРАТОР1/Модель турбины ==
  Generator speed (pu) : Inport
  Pitch angle (deg) : Inport  Port=2
  Wind speed (m/s) : Inport  Port=3
  Air density : Inport  Port=4
  1/cp_nom : Gain  Gain=1/cp_nom  SaturateOnIntegerOverflow=on  OutDataTypeStr=Inherit: Same as input  ParamDataTypeStr=Inherit: Same as input
  1/wind_base : Gain  Gain=1/wind_base  SaturateOnIntegerOverflow=on  OutDataTypeStr=Inherit: Same as input  ParamDataTypeStr=Inherit: Same as input
  Avoid division by zero : Saturate  UpperLimit=1e6  LowerLimit=1e-6
  "Avoid division by zero " : Saturate  UpperLimit=1e6  LowerLimit=1e-6
  Gain : Gain  Gain=-1  SaturateOnIntegerOverflow=on  OutDataTypeStr=Inherit: Same as input  ParamDataTypeStr=Inherit: Same as input
  Product : Product  Inputs=/*  SaturateOnIntegerOverflow=on  OutDataTypeStr=Inherit: Same as first input
  "Product " : Product  Inputs=3  SaturateOnIntegerOverflow=on  OutDataTypeStr=Inherit: Same as first input
  Product2 : Product  Inputs=*/  SaturateOnIntegerOverflow=on  InputSameDT=on  OutDataTypeStr=Inherit: Same as first input
  Saturation1 : Saturate  UpperLimit=inf  LowerLimit=1e-6
  Scope : Scope
  cp(lambda,beta) : Subsystem
  lambda_nom : Gain  Gain=lambda_nom  SaturateOnIntegerOverflow=on  OutDataTypeStr=Inherit: Same as input  ParamDataTypeStr=Inherit: Same as input
  pu->pu : Gain  Gain=P_wind_base*Pnom/Pelec_base  SaturateOnIntegerOverflow=on  OutDataTypeStr=Inherit: Same as input  ParamDataTypeStr=Inherit: Same as input
  "pu->pu " : Gain  Gain=1/speed_nom  SaturateOnIntegerOverflow=on  OutDataTypeStr=Inherit: Same as input  ParamDataTypeStr=Inherit: Same as input
  wind_speed^3 : Fcn  Expr=u(1)^3
  Tm (pu) : Outport  VectorParamsAs1DForOutWhenUnconnected=off
  wires:
  Pitch angle (deg)/1 -> cp(lambda,beta)/2(beta)
  pu->pu/1 -> Product2/1
  cp(lambda,beta)/1(cp) -> 1/cp_nom/1
  wind_speed^3/1 -> "Product "/1  "Pwind_pu"
  Product2/1 -> Gain/1
  Avoid division by zero/1 -> Product2/2
  Wind speed (m/s)/1 -> 1/wind_base/1
  Gain/1 -> Tm (pu)/1
  Generator speed (pu)/1 -> Avoid division by zero/1, "pu->pu "/1
  "Product "/1 -> pu->pu/1  "Pm_pu"
  lambda_nom/1 -> Saturation1/1  "lambda"
  1/cp_nom/1 -> "Product "/2  "cp_pu"
  Saturation1/1 -> cp(lambda,beta)/1(lambda), Scope/1
  Product/1 -> lambda_nom/1  "lambda_pu"
  1/wind_base/1 -> wind_speed^3/1, "Avoid division by zero "/1  "wind_speed_pu"
  "Avoid division by zero "/1 -> Product/1
  "pu->pu "/1 -> Product/2
  Air density/1 -> "Product "/3

== system WindPrototipeN/Дом 3/ВЕТРОТУРБИНА И ГЕНЕРАТОР1/Расчет номинального момента ==
  ПВ : Inport
  ОП : Inport  Port=2
  Base Torque : Product  Inputs=*/  RndMeth=Zero
  Base_torque_ : Display
  Constant1 : Constant  Value=8500
  Constant2 : Constant  Value=152.89
  Manual Switch1 : ManualSwitch  CurrentSetting=0
  Mux : Mux  Inputs=6
  Корректирующий коэффициент1 : Constant  Value=.0000133
  Коэффициент эффективности : Constant  Value=.43
  Номинальная мощность Вт : Constant  Value=2200
  Номинальная скорость ветра : Constant  Value=10
  Расчет номинального момента : Fcn  Expr=1/2*u(1)*u(2)*u(3)*u(4)^3*u(5)*u(6)
  Номинальный момент : Outport  VectorParamsAs1DForOutWhenUnconnected=off
  r : Outport  Port=2  VectorParamsAs1DForOutWhenUnconnected=off
  wires:
  Constant1/1 -> Base Torque/1
  ОП/1 -> Mux/2
  Расчет номинального момента/1 -> Manual Switch1/2, Base_torque_/1
  Коэффициент эффективности/1 -> Mux/3
  Номинальная скорость ветра/1 -> Mux/4
  Корректирующий коэффициент1/1 -> Mux/5
  Mux/1 -> Расчет номинального момента/1
  Номинальная мощность Вт/1 -> Mux/6
  Constant2/1 -> Manual Switch1/1
  Manual Switch1/1 -> r/1, Base Torque/2
  ПВ/1 -> Mux/1
  Base Torque/1 -> Номинальный момент/1

== system WindPrototipeN/Дом 3/ВХОДНЫЕ ЗНАЧЕНИЯ ДЛЯ ВЭУ1/Задание кривой скорости ==
  Demux : Demux  Tag=STV Demux  Outputs=1
  FromWs : FromWorkspace  Tag=STV FromWs  VariableName=tuvar  SampleTime=0
      SigBuilderData=|
      | common.afterFinalStr = 'Extrapolate'
      | common.sampleTime = 0
      | dataSet.timeRange = [0 15]
      | dataSet.name = 'Group 1'
      | sbobj.Groups.Name = 'Group 1'
      | sbobj.Groups.Signals.Name = 'Signal 1'
      | sbobj.Groups.Signals.XData = [0 1.5 2 2.5 3 4 5 7 8 9 11 15]
      | sbobj.Groups.Signals.YData = [9.95 10.05 9.9 10.4 10.4 10.25 10.74 11.85 11.2 11.64 10.52 10.2]
      | sbobj.Groups.TimeRange = [0 15]
  Signal 1 : Outport  Tag=STV Outport  VectorParamsAs1DForOutWhenUnconnected=off
  wires:
  Demux/1 -> Signal 1/1
  FromWs/1 -> Demux/1

== system WindPrototipeN/Дом 3/ВХОДНЫЕ ЗНАЧЕНИЯ ДЛЯ ВЭУ1/Задание кривой скорости1 ==
  Demux : Demux  Tag=STV Demux  Outputs=1
  FromWs : FromWorkspace  Tag=STV FromWs  VariableName=tuvar  SampleTime=0
      SigBuilderData=|
      | common.afterFinalStr = 'Extrapolate'
      | common.sampleTime = 0
      | dataSet.timeRange = [0 15]
      | dataSet.name = 'Group 1'
      | sbobj.Groups.Name = 'Group 1'
      | sbobj.Groups.Signals.Name = 'Signal 1'
      | sbobj.Groups.Signals.XData = [0 1.5 2 2.5 3 4 5 7 8 9 11 15]
      | sbobj.Groups.Signals.YData = [11.1 11.6 11.9 12.12 11.88 11.32 11.98 11.6 12 11.56 11.26 12]
      | sbobj.Groups.TimeRange = [0 15]
  Signal 1 : Outport  Tag=STV Outport  VectorParamsAs1DForOutWhenUnconnected=off
  wires:
  Demux/1 -> Signal 1/1
  FromWs/1 -> Demux/1

== system WindPrototipeN/Дом 3/ВХОДНЫЕ ЗНАЧЕНИЯ ДЛЯ СЭС1/Задание кривой солнечной радиации ==
  Demux : Demux  Tag=STV Demux
  FromWs : FromWorkspace  Tag=STV FromWs  VariableName=tuvar  SampleTime=0
      SigBuilderData=|
      | common.afterFinalStr = 'Extrapolate'
      | common.sampleTime = 0
      | dataSet.timeRange = [0 15]
      | dataSet.name = 'Group 1'
      | sbobj.Groups.Name = 'Group 1'
      | sbobj.Groups.Signals(1).Name = 'Signal 1'
      | sbobj.Groups.Signals(1).XData = [0 1 5 8 9 11 15]
      | sbobj.Groups.Signals(1).YData = [0 515 1190 1000 555 230 0]
      | sbobj.Groups.Signals(2).Name = 'Signal 2'
      | sbobj.Groups.Signals(2).XData = [0 2 2 3 3 15]
      | sbobj.Groups.Signals(2).YData = [0 0 1 1 0 0]
      | sbobj.Groups.Signals(3).Name = 'Signal 3'
      | sbobj.Groups.Signals(3).XData = [0 2.5 2.5 15]
      | sbobj.Groups.Signals(3).YData = [0 0 1 1]
      | sbobj.Groups.Signals(4).Name = 'Signal 4'
      | sbobj.Groups.Signals(4).XData = [0 2.5 2.5 15]
      | sbobj.Groups.Signals(4).YData = [0 0 1 1]
      | sbobj.Groups.TimeRange = [0 15]
  Signal 1 : Outport  Tag=STV Outport  VectorParamsAs1DForOutWhenUnconnected=off
  Signal 2 : Outport  Tag=STV Outport  Port=2
  Signal 3 : Outport  Tag=STV Outport  Port=3
  Signal 4 : Outport  Tag=STV Outport  Port=4
  wires:
  Demux/1 -> Signal 1/1
  FromWs/1 -> Demux/1
  Demux/2 -> Signal 2/1
  Demux/3 -> Signal 3/1
  Demux/4 -> Signal 4/1

== system WindPrototipeN/Дом 3/КОНТРОЛЛЕР БАТАРЕИ/Discrete PI Controller ==
  Error : Inport
  Discrete-Time Integrator : DiscreteIntegrator  InitialCondition=Init  SampleTime=Ts  LimitOutput=on  UpperSaturationLimit=UpperLimit  LowerSaturationLimit=LowerLimit  ICPrevOutput=DiscIntNeverNeededParam  ICPrevScaledInput=DiscIntNeverNeededParam
  Kp4 : Gain  Gain=Kp  SaturateOnIntegerOverflow=on  OutDataTypeStr=Inherit: Same as input  ParamDataTypeStr=Inherit: Same as input
  Kp5 : Gain  Gain=Ki  SaturateOnIntegerOverflow=on  OutDataTypeStr=Inherit: Same as input  ParamDataTypeStr=Inherit: Same as input
  Saturation2 : Saturate  UpperLimit=UpperLimit  LowerLimit=LowerLimit
  Sum6 : Sum  SaturateOnIntegerOverflow=on  InputSameDT=on  OutDataTypeStr=Inherit: Same as first input
  Out : Outport  InitialOutput=0  VectorParamsAs1DForOutWhenUnconnected=off
  wires:
  Saturation2/1 -> Out/1
  Discrete-Time Integrator/1 -> Sum6/2
  Kp4/1 -> Sum6/1
  Kp5/1 -> Discrete-Time Integrator/1
  Sum6/1 -> Saturation2/1
  Error/1 -> Kp5/1, Kp4/1

== system WindPrototipeN/Дом 3/КОНТРОЛЛЕР БАТАРЕИ/Discrete PI Controller1 ==
  Error : Inport
  Discrete-Time Integrator : DiscreteIntegrator  InitialCondition=Init  SampleTime=Ts  LimitOutput=on  UpperSaturationLimit=UpperLimit  LowerSaturationLimit=LowerLimit  ICPrevOutput=DiscIntNeverNeededParam  ICPrevScaledInput=DiscIntNeverNeededParam
  Kp4 : Gain  Gain=Kp  SaturateOnIntegerOverflow=on  OutDataTypeStr=Inherit: Same as input  ParamDataTypeStr=Inherit: Same as input
  Kp5 : Gain  Gain=Ki  SaturateOnIntegerOverflow=on  OutDataTypeStr=Inherit: Same as input  ParamDataTypeStr=Inherit: Same as input
  Saturation2 : Saturate  UpperLimit=UpperLimit  LowerLimit=LowerLimit
  Sum6 : Sum  SaturateOnIntegerOverflow=on  InputSameDT=on  OutDataTypeStr=Inherit: Same as first input
  Out : Outport  InitialOutput=0  VectorParamsAs1DForOutWhenUnconnected=off
  wires:
  Saturation2/1 -> Out/1
  Discrete-Time Integrator/1 -> Sum6/2
  Kp4/1 -> Sum6/1
  Kp5/1 -> Discrete-Time Integrator/1
  Sum6/1 -> Saturation2/1
  Error/1 -> Kp5/1, Kp4/1

== system WindPrototipeN/Дом 3/КОНТРОЛЛЕР БАТАРЕИ/Ramp_generator ==
  note: Carrier Freq
  Constant3 : Constant
  Discrete-Time Integrator1 : DiscreteIntegrator  ExternalReset=rising  SampleTime=20e-6  ICPrevOutput=DiscIntNeverNeededParam  ICPrevScaledInput=DiscIntNeverNeededParam
  Relational Operator1 : RelationalOperator  RndMeth=Nearest  InputSameDT=on
  Unit Delay1 : UnitDelay  SampleTime=20e-6  HasFrameUpgradeWarning=on
  fc : Constant  Value=10000
  ramp_out : Outport  VectorParamsAs1DForOutWhenUnconnected=off
  wires:
  Unit Delay1/1 -> Discrete-Time Integrator1/2
  Relational Operator1/1 -> Unit Delay1/1
  Constant3/1 -> Relational Operator1/2
  Discrete-Time Integrator1/1 -> ramp_out/1, Relational Operator1/1
  fc/1 -> Discrete-Time Integrator1/1

== system WindPrototipeN/Дом 3/ПОТРЕБИТЕЛЬ1/Subsystem1 ==
  Logical Operator{,1..3} (4 alike) : Logic  AllPortsSameDT=off  OutDataTypeStr=boolean
  Subsystem : Subsystem
  Кривая потребления : Subsystem  Tag=STV Subsys  LoadFcn=sigbuilder_block('load');  StartFcn=sigbuilder_block('start');  StopFcn=sigbuilder_block('stop');  ClipboardFcn=sigbuilder_block('clipboard');  mask(Sigbuilder block){tuvar=[0:10]}
      mask help: Simulink:masks:SigbuilderBlock_MD
      mask init:
      | if ~strcmp(get_param(bdroot(gcbh),'SimulationStatus'),'stopped') tuvar = sigbuilder_block('maskInit'); end
      settings: CopyFcn=sigbuilder_block('copy');  DeleteFcn=sigbuilder_block('delete');  ModelCloseFcn=sigbuilder_block('modelClose');  PreSaveFcn=sigbuilder_block('preSave');  PauseFcn=sigbuilder_block('pause');  ContinueFcn=sigbuilder_block('continue');  NameChangeFcn=sigbuilder_block('namechange');  OpenFcn=sigbuilder_block('open',[142.5 191.25 550.5 399.75 ]);  CloseFcn=sigbuilder_block('close');
      mask Display: plot(0, 0, 100, 100,[2, 2, 32, 32, 2], [68, 8, 8, 68, 68],[32, 2], [38, 38], [32, 19, 2],[53, 60, 44], [32, 17, 17, 2],[16, 16, 31, 31]);txt = getActiveGroup(gcbh);text(2, 100, txt,'verticalAlignment', 'top');
  Out1 : Outport
  Out2 : Outport  Port=2
  Out3 : Outport  Port=3
  Out4 : Outport  Port=4
  wires:
  Кривая потребления/4(Signal 4) -> Logical Operator3/2
  Subsystem/2(Out2) -> Logical Operator1/1
  Logical Operator/1 -> Out1/1
  Subsystem/4(Out4) -> Logical Operator3/1
  Subsystem/1(Out1) -> Logical Operator/1
  Кривая потребления/1(Signal 2) -> Logical Operator/2
  Кривая потребления/2(Signal 1) -> Logical Operator1/2
  Logical Operator2/1 -> Out3/1
  Кривая потребления/3(Signal 3) -> Logical Operator2/2
  Subsystem/3(Out3) -> Logical Operator2/1
  Logical Operator1/1 -> Out2/1
  Logical Operator3/1 -> Out4/1

== system WindPrototipeN/Дом 3/СОЛНЕЧНЫЕ ПАНЕЛИ1/11*2=666 V ==
  In1 : Inport
  Solar : Subsystem
  Conn1 : PMIOPort  Side=Right
  Conn2 : PMIOPort  Port=2  Side=Right
  wires:
  In1/1 -> Solar/1(In1)
  connections:
  Solar/RConn1 -- Conn1/RConn1
  Solar/RConn3 -- Solar/RConn2
  Conn2/RConn1 -- Solar/RConn4

== system WindPrototipeN/СИСТЕМА EMS/OPC/Subsystem ==
  In1 : Inport
  In2 : Inport  Port=2
  In3 : Inport  Port=3
  Data Type Conversion : DataTypeConversion  OutDataTypeStr=int8
  Data Type Conversion1 : DataTypeConversion  OutDataTypeStr=int8
  Data Type Conversion2 : DataTypeConversion  OutDataTypeStr=int8
  Out1 : Outport
  Out2 : Outport  Port=2
  Out3 : Outport  Port=3
  wires:
  In1/1 -> Data Type Conversion/1
  In2/1 -> Data Type Conversion1/1
  In3/1 -> Data Type Conversion2/1
  Data Type Conversion2/1 -> Out3/1
  Data Type Conversion1/1 -> Out2/1
  Data Type Conversion/1 -> Out1/1

== system WindPrototipeN/СИСТЕМА EMS/Измерение параметров виртуальной станции 1/Subsystem1 ==
  In1 : Inport
  Constant : Constant  Value=0
  IsNegative : simulink/Logic and Bit Operations/Compare To Zero  relop=<  OutDataTypeStr=boolean
  Switch : Switch
  Out1 : Outport
  wires:
  Constant/1 -> Switch/1
  In1/1 -> IsNegative/1, Switch/3
  Switch/1 -> Out1/1
  IsNegative/1 -> Switch/2

== system WindPrototipeN/СИСТЕМА EMS/Измерение параметров виртуальной станции 1/Subsystem2 ==
  In1 : Inport
  Constant : Constant  Value=0
  IsNegative : simulink/Logic and Bit Operations/Compare To Zero  relop=<  OutDataTypeStr=boolean
  Switch : Switch
  Out1 : Outport
  wires:
  Constant/1 -> Switch/1
  In1/1 -> IsNegative/1, Switch/3
  Switch/1 -> Out1/1
  IsNegative/1 -> Switch/2

== system WindPrototipeN/СИСТЕМА EMS/станция 2/Subsystem1 ==
  In1 : Inport
  Constant : Constant  Value=0
  IsNegative : simulink/Logic and Bit Operations/Compare To Zero  relop=<  OutDataTypeStr=boolean
  Switch : Switch
  Out1 : Outport
  wires:
  Constant/1 -> Switch/1
  In1/1 -> IsNegative/1, Switch/3
  Switch/1 -> Out1/1
  IsNegative/1 -> Switch/2

== system WindPrototipeN/СИСТЕМА EMS/станция 2/Subsystem2 ==
  In1 : Inport
  Constant : Constant  Value=0
  IsNegative : simulink/Logic and Bit Operations/Compare To Zero  relop=<  OutDataTypeStr=boolean
  Switch : Switch
  Out1 : Outport
  wires:
  Constant/1 -> Switch/1
  In1/1 -> IsNegative/1, Switch/3
  Switch/1 -> Out1/1
  IsNegative/1 -> Switch/2

== system WindPrototipeN/СИСТЕМА EMS/станция 3/Subsystem1 ==
  In1 : Inport
  Constant : Constant  Value=0
  IsNegative : simulink/Logic and Bit Operations/Compare To Zero  relop=<  OutDataTypeStr=boolean
  Switch : Switch
  Out1 : Outport
  wires:
  Constant/1 -> Switch/1
  In1/1 -> IsNegative/1, Switch/3
  Switch/1 -> Out1/1
  IsNegative/1 -> Switch/2

== system WindPrototipeN/СИСТЕМА EMS/станция 3/Subsystem2 ==
  In1 : Inport
  Constant : Constant  Value=0
  IsNegative : simulink/Logic and Bit Operations/Compare To Zero  relop=<  OutDataTypeStr=boolean
  Switch : Switch
  Out1 : Outport
  wires:
  Constant/1 -> Switch/1
  In1/1 -> IsNegative/1, Switch/3
  Switch/1 -> Out1/1
  IsNegative/1 -> Switch/2
